simulink model "impedance_subsystem"  (R2023a)
settings: Solver=VariableStepAuto  StartTime=0.0  StopTime=3  RelTol=1e-3
model workspace (MATLAB code in the model file):
  | %% Model component value calculations.
  | % Script recieves Thiele and Small values from mask and then calculates model components' values. It also stores values for sine sweep,
  | % A custom/manual sine sweep was needed inorder to get values for the variable resistors.
  | 
  | Re=         [str2double(get_param('a_LS_model/T&S Values', 'W_Re')), str2double(get_param('a_LS_model/T&S Values', 'T_Re'))];           % The DC resistance of the Voice coil [ohm].
  | 
  | Le=         [str2double(get_param('a_LS_model/T&S Values', 'W_Le')), str2double(get_param('a_LS_model/T&S Values', 'T_Le'))] *1e-3; % The voice coil inductance [H]
  | 
  | 
  | Mms=        [str2double(get_param('a_LS_model/T&S Values', 'W_Mms')), str2double(get_param('a_LS_model/T&S Values', 'T_Mms'))]    *1e-3;  % Mass of the coil and diagphram [Kg]
  | 
  | Sd=         [str2double(get_param('a_LS_model/T&S Values', 'W_Sd')), str2double(get_param('a_LS_model/T&S Values', 'T_Sd'))]    *1e-4;  %Area of diagphram [m^2]
  | Bl=      [str2double(get_param('a_LS_model/T&S Values', 'W_Bl')), str2double(get_param('a_LS_model/T&S Values', 'T_Bl'))];            %The product of magnetic flux density ie Force Factor
  | Vb = [str2double(get_param('a_LS_model/T&S Values', 'Vb')),str2double(get_param('a_LS_model/T&S Values', 'Vb'))];
  | fs =[str2double(get_param('a_LS_model/T&S Values', 'W_fs')),str2double(get_param('a_LS_model/T&S Values', 'T_fs'))];
  | Qes = [str2double(get_param('a_LS_model/T&S Values', 'W_Qes')),str2double(get_param('a_LS_model/T&S Values', 'T_Qes'))];
  | Qms = [str2double(get_param('a_LS_model/T&S Values', 'W_Qms')),str2double(get_param('a_LS_model/T&S Values', 'T_Qms'))];
  | Qts = [str2double(get_param('a_LS_model/T&S Values', 'W_Qts')),str2double(get_param('a_LS_model/T&S Values', 'T_Qts'))];
  | 
  | SweepStart_W_S =str2double(get_param('a_LS_model/Subsystem4', 'SweepStart'));
  | SweepEnd_W_S = str2double(get_param('a_LS_model/Subsystem4', 'SweepStop'));
  | SweepDuration_W_S =str2double(get_param('a_LS_model/Subsystem4', 'SweepTime'));
  | 
  | Vb = Vb ./ 1000;
  | FS = 44100;
  | Qb = 0.707; % Total quality factor
  | 
  | % Constants
  | c = 340; % Speed of sound in m/s
  | rho = 1.2; % Density of air [kg/m^3]
  | 
  | for n = 1:2
  |     alpha(n) = (Qb^2 - Qts(n)^2) / Qts(n)^2;
  |     Rms(n) = (2 * pi * fs(n) * Mms(n)) / Qms(n);
  |     Cms(n) = 1 / (4 * pi^2 * fs(n)^2 * Mms(n));
  |     Vas(n)=rho*c*Sd(n)^2*Cms(n);
  | end
  | 
  | QB = sqrt(alpha(1) + 1) * Qts; % Electroacostics Lecture 4 page 21
  | 
  | for n = 1:2
  | 
  |     r=0.1;
  |     Cab(n) = Vb(n) / (rho * c^2); % Box volume acoustic compliance
  | 
  |     a(n) = sqrt(Sd(n) / pi);
  |     a(n) = 0.85
  |     %Zc(n) = ((rho * c) / Sd(n)) * c; % from grain42n
  | 
  |     Mad(n) = (8 * rho) / (5 * (pi^2) * a(n));% Mad (acoustic mass)
  |     Mar(n)=rho*((a(n)*r)/Sd(n)) % from grain42n
  |     Mad(n)=Mar(n);
  |     Ras(n) = (rho * c) / (pi * (a(n)^2)); %  Ras (acoustic resistance), Beranek page 820/ grain42-page 19
  | 
  |     Lem(n) = Bl(n)^2 * Cms(n); % Lem (driver's equivalent inductance)
  |     Rem(n) = Bl(n)^2 / Rms(n); % Rem (driver's equivalent mechanical resistance),
  |     Cem(n) = Mms(n) / (Bl(n)^2); % Cem (driver's equivalent compliance) from grain41en
  | 
  |     Leb(n) = (Bl(n)/Sd(n))^2 *Cab(n);% Lea (acoustical inductance) grain42-page 19
  |     Rer(n) = (Bl(n)/Sd(n))^2 * 1/Ras(n); % Rea (acoustical resistance)
  |     Cer(n) = (Sd(n)/Bl(n))^2 *Mar(n);%Cea (acoustical compliance
  |     Ced(n) = (Sd(n)/Bl(n))^2 * Mad(n);% Borwick Headphones page 304
  | 
  | end
undefined symbols (not defined in the file): Ced, Cem, Cer, Leb, Lem, Rem
libraries: fl_lib x29, nesl_utility x12, dspsrcs4 x1
settings Model: Creator=Jamie  LastModifiedBy=jamie

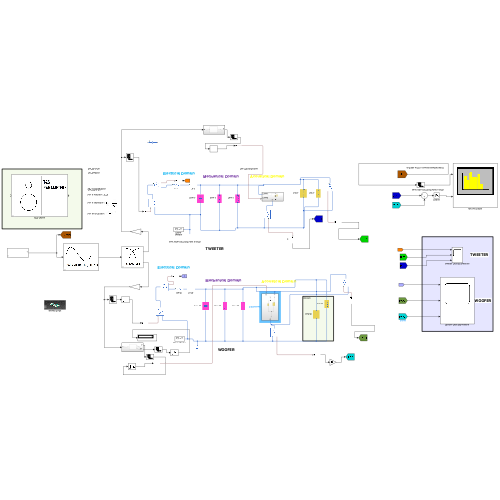
[thumbnail: Simulink's stored preview of the top-level diagram]
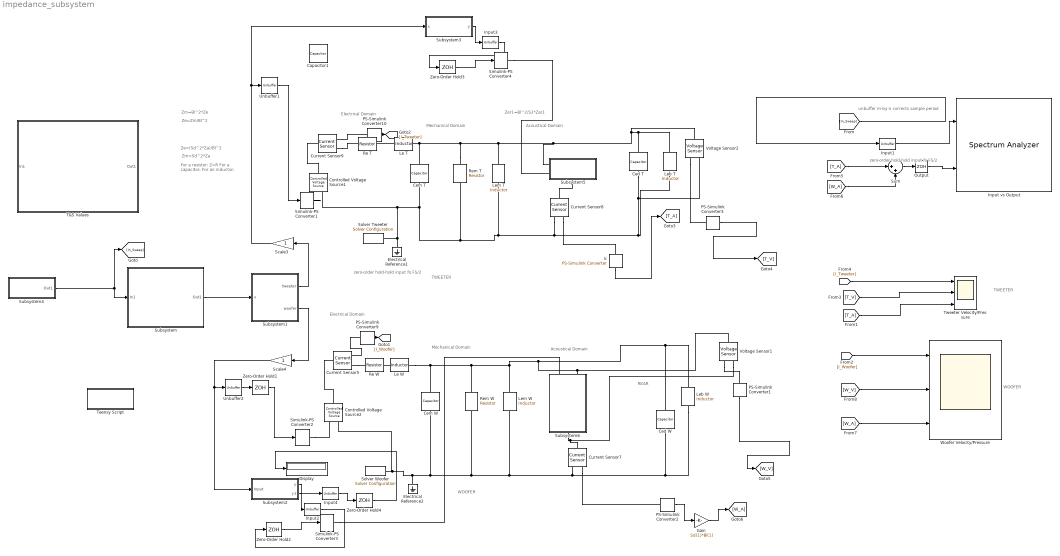
== system impedance_subsystem ==
  note: Zer1=Bl^2/S2*Zar1
  note: Electrical Domain
  note: Mechanical Domain
  note: Mechanical Domain
  note: Zm=Bl^2*Ze
  note: WOOFER
  note: WOOFER
  note: unbuffer m-by-n corrects sample period
  note: TWEETER
  note: Acoustical Domain
  note: zero-order hold-hold input fo FS/2
  note: Zm=Sd^2*Za
  note: For a resistor: Z=R
      | For a capacitor:
      | For an inductor:
  note: zero-order hold-hold input fo FS/2
  note: Ze=Zm/Bl^2
  note: TWEETER
  note: Ze=(Sd^2*Za)/Bl^2
  note: Electrical Domain
  note: Acoustical Domain
  note: REAR
  Capacitor1 : fl_lib/Electrical/Electrical Elements/Capacitor  c=1000 uF  r=1e-6 Ohm  g=0 1/Ohm  i_specify=off  i_priority=None  i=0 A  i_nominal_specify=off  i_nominal_unit=A  i_nominal_value=1  v_specify=off  v_priority=None  v=0 V  v_nominal_specify=off  v_nominal_unit=V  v_nominal_value=1  vc_specify=off  vc_priority=High  vc=0 V  vc_nominal_specify=off  vc_nominal_unit=V  vc_nominal_value=1
  Ced T : fl_lib/Electrical/Electrical Elements/Capacitor  c=Ced(2) F  r=0 Ohm  g=0 1/Ohm  i_specify=off  i_priority=High  i=0 A  i_nominal_specify=off  i_nominal_unit=A  i_nominal_value=1  v_specify=off  v_priority=High  v=0 V  v_nominal_specify=off  v_nominal_unit=V  v_nominal_value=1  vc_specify=off  vc_priority=High  vc=0 V  vc_nominal_specify=off  vc_nominal_unit=V  vc_nominal_value=1
  Ced W : fl_lib/Electrical/Electrical Elements/Capacitor  c=Ced(1) F  r=0 Ohm  g=0 1/Ohm  i_specify=off  i_priority=High  i=0 A  i_nominal_specify=off  i_nominal_unit=A  i_nominal_value=1  v_specify=off  v_priority=High  v=0 V  v_nominal_specify=off  v_nominal_unit=V  v_nominal_value=1  vc_specify=off  vc_priority=High  vc=0 V  vc_nominal_specify=off  vc_nominal_unit=V  vc_nominal_value=1
  Cem T : fl_lib/Electrical/Electrical Elements/Capacitor  c=Cem(2) F  r=0 Ohm  g=0 1/Ohm  i_specify=off  i_priority=High  i=0 A  i_nominal_specify=off  i_nominal_unit=A  i_nominal_value=1  v_specify=off  v_priority=High  v=0 V  v_nominal_specify=off  v_nominal_unit=V  v_nominal_value=1  vc_specify=off  vc_priority=High  vc=0 V  vc_nominal_specify=off  vc_nominal_unit=V  vc_nominal_value=1
  Cem W : fl_lib/Electrical/Electrical Elements/Capacitor  c=Cem(1) F  r=0 Ohm  g=0 1/Ohm  i_specify=off  i_priority=High  i=0 A  i_nominal_specify=off  i_nominal_unit=A  i_nominal_value=1  v_specify=off  v_priority=High  v=0 V  v_nominal_specify=off  v_nominal_unit=V  v_nominal_value=1  vc_specify=off  vc_priority=High  vc=0 V  vc_nominal_specify=off  vc_nominal_unit=V  vc_nominal_value=1
  Controlled Voltage Source1 : fl_lib/Electrical/Electrical Sources/Controlled Voltage Source
  Controlled Voltage Source2 : fl_lib/Electrical/Electrical Sources/Controlled Voltage Source
  Current Sensor{5,7..9} (4 alike) : fl_lib/Electrical/Electrical Sensors/Current Sensor
  Display : Display
  Electrical Reference1 : fl_lib/Electrical/Electrical Elements/Electrical Reference
  Electrical Reference2 : fl_lib/Electrical/Electrical Elements/Electrical Reference
  Gain : Gain  Gain=Sd(1)*Bl(1)
  "Input vs Output " : SpectrumAnalyzer  NumInputPorts=2  WindowPosition=[115.000000,110.000000,1536.000000,801.000000,]  ScopeFrameLocation=window  SpectrumType=Power density  Method=Welch  SampleRate=48000  PlotAsTwoSidedSpectrum=off  FrequencyScale=Log  AxesScaling=Manual  FrequencySpan=Start and stop frequencies  StartFrequency=4000  StopFrequency=20e3  AveragingMethod=Exponential  ForgettingFactor=0.4  SpectrumUnits=dBm/Hz  PlotMaxHoldTrace=on  YLimits=[-240.83457972,36.18497741]  ShowLegend=on  SelectedToolstripTab=spectrumAnalyzerToolstrip.spectrumTab  MeasurementChannel=4
      settings: OpenAtSimulationStart=off
  Input{1..4} (4 alike) : Unbuffer
  Le T : fl_lib/Electrical/Electrical Elements/Inductor  l=Le(2) H  r=0 Ohm  g=0 1/Ohm  i_specify=off  i_priority=High  i=0 A  i_nominal_specify=off  i_nominal_unit=A  i_nominal_value=1  v_specify=off  v_priority=High  v=0 V  v_nominal_specify=off  v_nominal_unit=V  v_nominal_value=1  i_L_specify=off  i_L_priority=High  i_L=0 A  i_L_nominal_specify=off  i_L_nominal_unit=A  i_L_nominal_value=1
  Le W : fl_lib/Electrical/Electrical Elements/Inductor  l=Le(1) H  r=0 Ohm  g=0 1/Ohm  i_specify=off  i_priority=High  i=0 A  i_nominal_specify=off  i_nominal_unit=A  i_nominal_value=1  v_specify=off  v_priority=High  v=0 V  v_nominal_specify=off  v_nominal_unit=V  v_nominal_value=1  i_L_specify=off  i_L_priority=High  i_L=0 A  i_L_nominal_specify=off  i_L_nominal_unit=A  i_L_nominal_value=1
  Leb T : fl_lib/Electrical/Electrical Elements/Inductor  l=Leb(2) H  r=0 Ohm  g=0 1/Ohm  i_specify=off  i_priority=High  i=0 A  i_nominal_specify=off  i_nominal_unit=A  i_nominal_value=1  v_specify=off  v_priority=High  v=0 V  v_nominal_specify=off  v_nominal_unit=V  v_nominal_value=1  i_L_specify=off  i_L_priority=High  i_L=0 A  i_L_nominal_specify=off  i_L_nominal_unit=A  i_L_nominal_value=1
  Leb W : fl_lib/Electrical/Electrical Elements/Inductor  l=Leb(1) H  r=0 Ohm  g=0 1/Ohm  i_specify=off  i_priority=High  i=0 A  i_nominal_specify=off  i_nominal_unit=A  i_nominal_value=1  v_specify=off  v_priority=High  v=0 V  v_nominal_specify=off  v_nominal_unit=V  v_nominal_value=1  i_L_specify=off  i_L_priority=High  i_L=0 A  i_L_nominal_specify=off  i_L_nominal_unit=A  i_L_nominal_value=1
  Lem T : fl_lib/Electrical/Electrical Elements/Inductor  l=Lem(2) H  r=0 Ohm  g=0 1/Ohm  i_specify=off  i_priority=High  i=0 A  i_nominal_specify=off  i_nominal_unit=A  i_nominal_value=1  v_specify=off  v_priority=High  v=0 V  v_nominal_specify=off  v_nominal_unit=V  v_nominal_value=1  i_L_specify=off  i_L_priority=High  i_L=0 A  i_L_nominal_specify=off  i_L_nominal_unit=A  i_L_nominal_value=1
  Lem W : fl_lib/Electrical/Electrical Elements/Inductor  l=Lem(1) H  r=0 Ohm  g=0 1/Ohm  i_specify=off  i_priority=High  i=0 A  i_nominal_specify=off  i_nominal_unit=A  i_nominal_value=1  v_specify=off  v_priority=High  v=0 V  v_nominal_specify=off  v_nominal_unit=V  v_nominal_value=1  i_L_specify=off  i_L_priority=High  i_L=0 A  i_L_nominal_specify=off  i_L_nominal_unit=A  i_L_nominal_value=1
  Output : ZeroOrderHold  SampleTime=1/FS
  PS-Simulink Converter{1..3,9..10} (5 alike) : nesl_utility/PS-Simulink Converter  PhysicalDomain=network_engine_domain  SubClassName=ps_output  LeftPortType=input  RightPortType=output  PseudoPeriodic=off  Frequencies=[]  VectorFormat=1-D array  Unit=1  AffineConversion=off
  Re T : fl_lib/Electrical/Electrical Elements/Resistor  R=Re(2) Ohm  i_specify=off  i_priority=High  i=0 A  i_nominal_specify=off  i_nominal_unit=A  i_nominal_value=1  v_specify=off  v_priority=High  v=0 V  v_nominal_specify=off  v_nominal_unit=V  v_nominal_value=1
  Re W : fl_lib/Electrical/Electrical Elements/Resistor  R=Re(1) Ohm  i_specify=off  i_priority=High  i=0 A  i_nominal_specify=off  i_nominal_unit=A  i_nominal_value=1  v_specify=off  v_priority=High  v=0 V  v_nominal_specify=off  v_nominal_unit=V  v_nominal_value=1
  Rem T : fl_lib/Electrical/Electrical Elements/Resistor  R=Rem(2) Ohm  i_specify=off  i_priority=High  i=0 A  i_nominal_specify=off  i_nominal_unit=A  i_nominal_value=1  v_specify=off  v_priority=High  v=0 V  v_nominal_specify=off  v_nominal_unit=V  v_nominal_value=1
  Rem W : fl_lib/Electrical/Electrical Elements/Resistor  R=Rem(1) Ohm  i_specify=off  i_priority=High  i=0 A  i_nominal_specify=off  i_nominal_unit=A  i_nominal_value=1  v_specify=off  v_priority=High  v=0 V  v_nominal_specify=off  v_nominal_unit=V  v_nominal_value=1
  Scale3 : Gain
  Scale4 : Gain
  Simulink-PS Converter{1..4} (4 alike) : nesl_utility/Simulink-PS Converter  PhysicalDomain=network_engine_domain  SubClassName=ps_input  LeftPortType=input  RightPortType=output  PseudoPeriodic=off  Frequencies=[]  NoiseDistribution=none  NoiseParameters=[]  Unit=1  AffineConversion=off  FilteringAndDerivatives=zero  SimscapeFilterOrder=1  InputFilterTimeConstant=0.001  UdotUserProvided=1
  Solver Tweeter : nesl_utility/Solver Configuration  PhysicalDomain=network_engine_domain  SubClassName=solver  LeftPortType=input  RightPortType=generic  Tones=[]  Harmonics=[]  SimulateNoise=off  Profile=off  UseLocalSampling=off  EnableSwitchedLinearOptims=on  FrequencyDomain=off  UseCCode=off  RelTol=0.001  AbsTol=1e-06  MinStep=1e-09  ToWorkspace=off  RevertToSquareIcSolve=off  NumHomotopyIterations=100  PhasorMode=off  PhasorModeNumHarmonics=1  ConsistencySolver=NEWTON_FTOL  IndexReductionMethod=DerivativeReplacement  DoDC=off  ResidualTolerance=1e-09  ConsistencyTolSource=GLOBAL  ConsistencyAbsTol=0.001  ConsistencyRelTol=0.001  ConsistencyTolFactor=0.001  UseLocalSolver=off  LocalSolverChoice=NE_BACKWARD_EULER_ADVANCER  ResolveIndetEquations=on  FunctionEvalNumThread=1  LocalSolverSampleTime=0.001  DoFixedCost=off  MaxNonlinIter=3  MaxModeIter=2  ComputeImpulses=off  ImpulseIterations=2  LinearAlgebra=Sparse  LinearAlgebraNumThread=0  EquationFormulation=NE_TIME_EF  DelaysMemoryBudget=1024  AutomaticFiltering=on  FilteringTimeConstant=0.001  PartitionStorageMethod=AS_NEEDED  PartitionMemoryBudget=1024  PartitionMethod=FAST
  "Solver Woofer " : nesl_utility/Solver Configuration  PhysicalDomain=network_engine_domain  SubClassName=solver  LeftPortType=input  RightPortType=generic  Tones=[]  Harmonics=[]  SimulateNoise=off  Profile=off  UseLocalSampling=off  EnableSwitchedLinearOptims=on  FrequencyDomain=off  UseCCode=off  RelTol=0.001  AbsTol=1e-06  MinStep=1e-09  ToWorkspace=off  RevertToSquareIcSolve=off  NumHomotopyIterations=100  PhasorMode=off  PhasorModeNumHarmonics=1  ConsistencySolver=NEWTON_FTOL  IndexReductionMethod=DerivativeReplacement  DoDC=off  ResidualTolerance=1e-09  ConsistencyTolSource=GLOBAL  ConsistencyAbsTol=0.001  ConsistencyRelTol=0.001  ConsistencyTolFactor=0.001  UseLocalSolver=off  LocalSolverChoice=NE_BACKWARD_EULER_ADVANCER  ResolveIndetEquations=on  FunctionEvalNumThread=1  LocalSolverSampleTime=0.001  DoFixedCost=off  MaxNonlinIter=3  MaxModeIter=2  ComputeImpulses=off  ImpulseIterations=2  LinearAlgebra=Sparse  LinearAlgebraNumThread=0  EquationFormulation=NE_TIME_EF  DelaysMemoryBudget=1024  AutomaticFiltering=on  FilteringTimeConstant=0.001  PartitionStorageMethod=AS_NEEDED  PartitionMemoryBudget=1024  PartitionMethod=FAST
  Subsystem : Subsystem  mask{plotFlag=on, BW1=88.120, GdB1=0, FC1=500, BW2=59.410, GdB2=0, FC2=1.352e+03, BW3=100.0, GdB3=0, FC3=400, BW4=67.330, GdB4=0, FC4=400, BW5=66.340, GdB5=0, FC5=129.131, BW6=53.470, GdB6=0, FC6=833.739}
      mask prompts: plotFlag "Plot EQ response"; BW1 "Band Width 1"; GdB1 "Gain 1"; FC1 "Center Frequency 1"; BW2 "Band Width 2"; GdB2 "Gain 2"; FC2 "Center Frequency 2"; BW3 "Band Width 3"; GdB3 "Gain 3"; FC3 "Center Frequency 3"; BW4 "Band Width 4"; GdB4 "Gain 4"; FC4 "Center Frequency 4"; BW5 "Band Width 5"; GdB5 "Gain 5"; FC5 "Center Frequency 5"; BW6 "Band Width 6"; GdB6 "Gain 6"; FC6 "Center Frequency 6"
      mask DialogControl DescTextVar Prompt: Highest and lowest fc will be shelving
      mask Display: image('parametric equalizer.jpg'); % Use "Edit Image" on toolstrip to change.
  Subsystem1 : Subsystem  mask{fc=1.069e+03, G_T=5.040, G_W=0, response=on}
      mask prompts: G_T "Tweeter Gain"; G_W "Wooofer Gain"; response "Plot frequency response"
      mask Display: image('crossover.jpg'); % Use "Edit Image" on toolstrip to change.
  Subsystem2 : Subsystem
  Subsystem3 : Subsystem
  Subsystem4 : Subsystem  mask{SweepStart=20.0, SweepStop=2.000e+04, SweepTime=3}
      mask prompts: SweepStart "Sweep start frequency"; SweepStop "Sweep end frequency"; SweepTime "Sweep time in seconds"
  Subsystem5 : Subsystem
      settings: PortSchema="{\"entries\":[{\"content\":{\"sides\":[{\"content\":{\"connectorIds\":[\"LConn1\",\"LConn2\"]},\"type\":\"ConnectorPlacement.EquallySpacedRectSide\",\"uuid\":\"25cb09ee-3296-462f-b9af-d61a9c9e7aa7\"},{\"content\":{\"side\":\"RIGHT\"},\"type\":\"ConnectorPlacement.EquallySpacedRectSide\",\"uuid\":\"56b7f4d6-4575-4235-9b40-81966edcf44f\"},{\"content\":{\"side\":\"TOP\"},\"type\":\"ConnectorPlacement.EquallySpacedRectSide\",\"uuid\":\"6b15c573-0474-440b-b33a-e36954ffc872\"},{\"content\":{\"connectorIds\":[\"RConn1\"],\"side\":\"BOTTOM\"},\"type\":\"ConnectorPlacement.EquallySpacedRectSide\",\"uuid\":\"46e98950-34e6-48c0-ad9b-f72df4e485f9\"}]},\"type\":\"ConnectorPlacement.EquallySpacedConnector\",\"uuid\":\"8a04249c-d482-4767-9f60-a5a89d31e022\"}],\"packageUris\":[\"http://schema.mathworks.com/mf0/Connector/R2020b\"],\"version\":\"1.0\"}"
  Subsystem6 : Subsystem
  Sum : Sum  Inputs=|++
  T&S Values : Subsystem  mask{Vb=1000, W_Sd=56.4, T_Sd=6.2, W_Re=3.7, T_Re=3.2, W_Le=0.22, T_Le=0.04, W_Bl=5, T_Bl=1.6, W_Mms=6.7, T_Mms=0.3, W_fs=74.6, T_fs=750, W_Qts=4.84, T_Qts=1.12, W_Qes=0.47, T_Qes=1.78, W_Qms=0.43, T_Qms=3.0}
      mask prompts: Vb "Box Volume"; W_Sd "Woofer Sd"; T_Sd "Tweeter Sd"; W_Re "Woofer Re"; T_Re "Tweeter Re"; W_Le "Woofer Le"; T_Le "Tweeter Le"; W_Bl "Woofer Bl"; T_Bl "Tweeter Bl"; W_Mms "Woofer Mms"; T_Mms "Tweeter Mms"; W_fs "Woofer fs"; T_fs "Tweeter fs"; W_Qts "Woofer Qts"; T_Qts "Tweeter Qts"; W_Qes "Woofer Qes"; T_Qes "Tweeter Qes"; W_Qms "Woofer Qms"; T_Qms "Tweeter Qms"
      mask Display: image('$imagefile'); % Use "Edit Image" on toolstrip to change.
  Teensy Script : Subsystem  mask{savename=modified_script2.txt}
      mask prompts: savename "Script.txt save name"
      mask Display: image('teensy_pic_for_mask.jpg'); % Use "Edit Image" on toolstrip to change.
  Tweeter Velocity/Pressure : Scope  NumInputPorts=3
  Unbuffer1 : Unbuffer
  Unbuffer2 : Unbuffer
  Voltage Sensor1 : fl_lib/Electrical/Electrical Sensors/Voltage Sensor
  Voltage Sensor2 : fl_lib/Electrical/Electrical Sensors/Voltage Sensor
  Woofer Velocity/Pressure : Scope  NumInputPorts=3
  Zero-Order Hold{1..4} (4 alike) : ZeroOrderHold  SampleTime=1/FS
  "k " : nesl_utility/PS-Simulink Converter  PhysicalDomain=network_engine_domain  SubClassName=ps_output  LeftPortType=input  RightPortType=output  PseudoPeriodic=off  Frequencies=[]  VectorFormat=1-D array  Unit=1  AffineConversion=off
  wires:
  Zero-Order Hold3/1 -> Simulink-PS Converter4/1
  Subsystem2/1(y) -> Input2/1
  Zero-Order Hold1/1 -> Simulink-PS Converter2/1
  [I_Tweeter] -> Tweeter Velocity/Pressure/1
  PS-Simulink Converter9/1 -> [I_Woofer]
  Subsystem3/1(y) -> Input3/1
  Input2/1 -> Zero-Order Hold2/1
  Subsystem1/2(woofer) -> Scale4/1
  Unbuffer2/1 -> Zero-Order Hold1/1
  Zero-Order Hold2/1 -> Simulink-PS Converter3/1
  PS-Simulink Converter3/1 -> [T_V]
  Input3/1 -> Zero-Order Hold3/1
  [I_Woofer] -> Woofer Velocity/Pressure/1
  [T_A] -> Sum/1
  PS-Simulink Converter10/1 -> [I_Tweeter]
  Subsystem4/1(Out1) -> [In_Sweep], Subsystem/1(In1)
  Sum/1 -> Output/1
  Unbuffer1/1 -> Simulink-PS Converter1/1
  Subsystem1/1(tweeter) -> Scale3/1
  "k "/1 -> [T_A]
  [W_A] -> Sum/2
  PS-Simulink Converter1/1 -> [W_V]
  Subsystem/1(Out1) -> Subsystem1/1(x)
  Subsystem2/2(y1) -> Input4/1
  Input4/1 -> Zero-Order Hold4/1
  Zero-Order Hold4/1 -> Display/1
  Input1/1 -> "Input vs Output "/1
  [In_Sweep] -> Input1/1
  Output/1 -> "Input vs Output "/2
  Scale3/1 -> Subsystem3/1(x), Unbuffer1/1
  Scale4/1 -> Subsystem2/1(Input), Unbuffer2/1
  PS-Simulink Converter2/1 -> Gain/1
  Gain/1 -> [W_A]
  [W_V] -> Woofer Velocity/Pressure/2
  [W_A] -> Woofer Velocity/Pressure/3
  [T_A] -> Tweeter Velocity/Pressure/3
  [T_V] -> Tweeter Velocity/Pressure/2
  connections:
  Rem T/LConn1 -- Cem T/LConn1 -- Le T/RConn1 -- Lem T/LConn1 -- Subsystem5/LConn1 -- Ced T/LConn1 -- Leb T/LConn1 -- Voltage Sensor2/LConn1
  Lem W/LConn1 -- Voltage Sensor1/LConn1 -- Subsystem6/LConn1 -- Ced W/LConn1 -- Leb W/LConn1 -- Rem W/LConn1 -- Cem W/LConn1 -- Le W/RConn1
  Voltage Sensor1/RConn1 -- PS-Simulink Converter1/LConn1
  Simulink-PS Converter1/RConn1 -- Controlled Voltage Source1/RConn1
  Simulink-PS Converter4/RConn1 -- Subsystem5/LConn2
  PS-Simulink Converter10/LConn1 -- Current Sensor9/RConn1
  Ced W/RConn1 -- Current Sensor7/RConn2 -- "Solver Woofer "/RConn1 -- Controlled Voltage Source2/RConn2 -- Electrical Reference2/LConn1 -- Cem W/RConn1 -- Rem W/RConn1 -- Lem W/RConn1 -- Leb W/RConn1
  Le W/LConn1 -- Re W/RConn1
  Current Sensor8/RConn1 -- "k "/LConn1
  Simulink-PS Converter2/RConn1 -- Controlled Voltage Source2/RConn1
  Simulink-PS Converter3/RConn1 -- Subsystem6/LConn2
  Le T/LConn1 -- Re T/RConn1
  Ced T/RConn1 -- Voltage Sensor2/RConn2 -- Current Sensor8/RConn2 -- Lem T/RConn1 -- Rem T/RConn1 -- Solver Tweeter/RConn1 -- Electrical Reference1/LConn1 -- Controlled Voltage Source1/RConn2 -- Cem T/RConn1 -- Leb T/RConn1
  PS-Simulink Converter9/LConn1 -- Current Sensor5/RConn1
  Voltage Sensor2/RConn1 -- PS-Simulink Converter3/LConn1
  Current Sensor7/RConn1 -- PS-Simulink Converter2/LConn1
  Current Sensor9/RConn2 -- Re T/LConn1
  Current Sensor9/LConn1 -- Controlled Voltage Source1/LConn1
  Controlled Voltage Source2/LConn1 -- Current Sensor5/LConn1
  Current Sensor5/RConn2 -- Re W/LConn1
  Subsystem5/RConn1 -- Current Sensor8/LConn1
  Subsystem6/RConn1 -- Current Sensor7/LConn1 -- Voltage Sensor1/RConn2

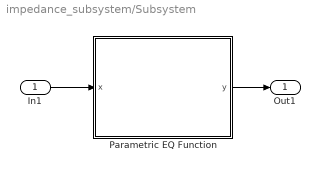
== system impedance_subsystem/Subsystem ==
  In1 : Inport
  Parametric EQ Function : MATLAB Function  TreatAsAtomicUnit=on
  Out1 : Outport
  wires:
  In1/1 -> Parametric EQ Function/1(x)
  Parametric EQ Function/1(y) -> Out1/1

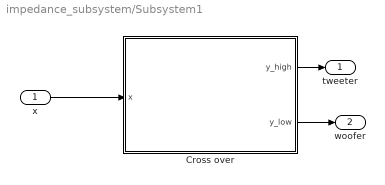
== system impedance_subsystem/Subsystem1 ==
  x : Inport
  Cross over : MATLAB Function  TreatAsAtomicUnit=on
  tweeter : Outport
  woofer : Outport  Port=2
  wires:
  x/1 -> Cross over/1(x)
  Cross over/1(y_high) -> tweeter/1
  Cross over/2(y_low) -> woofer/1

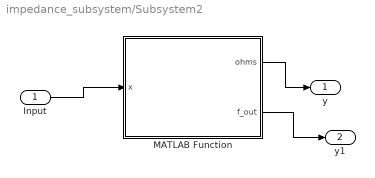
== system impedance_subsystem/Subsystem2 ==
  Input : Inport
  MATLAB Function : MATLAB Function  TreatAsAtomicUnit=on
  y : Outport
  y1 : Outport  Port=2
  wires:
  MATLAB Function/1(ohms) -> y/1
  MATLAB Function/2(f_out) -> y1/1
  Input/1 -> MATLAB Function/1(x)

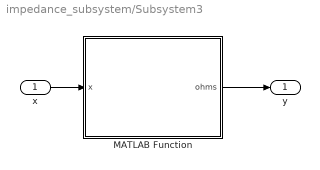
== system impedance_subsystem/Subsystem3 ==
  x : Inport
  MATLAB Function : MATLAB Function  TreatAsAtomicUnit=on
  y : Outport
  wires:
  x/1 -> MATLAB Function/1(x)
  MATLAB Function/1(ohms) -> y/1

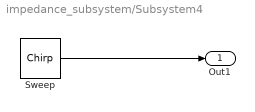
== system impedance_subsystem/Subsystem4 ==
  Sweep : dspsrcs4/Chirp  sweep=Logarithmic  mode=Unidirectional  f0=SweepStart  f1=SweepStop  t1=SweepTime  Tsweep=SweepTime  phase=0  Ts=1/FS  spf=1024  datatype=Double  OutputFrames=off
  Out1 : Outport
  wires:
  Sweep/1 -> Out1/1

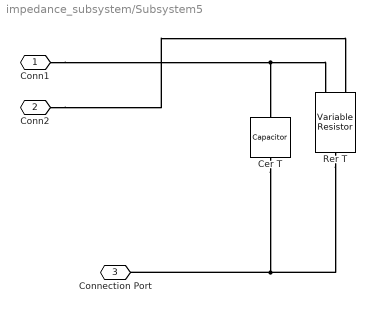
== system impedance_subsystem/Subsystem5 ==
  Cer T : fl_lib/Electrical/Electrical Elements/Capacitor  c=Cer(2) F  r=0 Ohm  g=0 1/Ohm  i_specify=off  i_priority=High  i=0 A  i_nominal_specify=off  i_nominal_unit=A  i_nominal_value=1  v_specify=off  v_priority=High  v=0 V  v_nominal_specify=off  v_nominal_unit=V  v_nominal_value=1  vc_specify=off  vc_priority=High  vc=0 V  vc_nominal_specify=off  vc_nominal_unit=V  vc_nominal_value=1
  Rer T : fl_lib/Electrical/Electrical Elements/Variable Resistor  Rmin=0 Ohm  i_specify=off  i_priority=None  i=0 A  i_nominal_specify=off  i_nominal_unit=A  i_nominal_value=1  v_specify=off  v_priority=None  v=0 V  v_nominal_specify=off  v_nominal_unit=V  v_nominal_value=1
  Conn1 : PMIOPort  Side=Left
  Conn2 : PMIOPort  Port=2  Side=Left
  Connection Port : PMIOPort  Port=3  Side=Right
  connections:
  Conn1/RConn1 -- Rer T/LConn2 -- Cer T/LConn1
  Cer T/RConn1 -- Rer T/RConn1 -- Connection Port/RConn1
  Conn2/RConn1 -- Rer T/LConn1

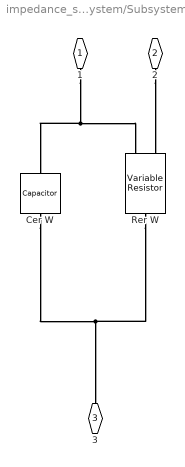
== system impedance_subsystem/Subsystem6 ==
  Cer W : fl_lib/Electrical/Electrical Elements/Capacitor  c=Cer(1) F  r=0 Ohm  g=0 1/Ohm  i_specify=off  i_priority=High  i=0 A  i_nominal_specify=off  i_nominal_unit=A  i_nominal_value=1  v_specify=off  v_priority=High  v=0 V  v_nominal_specify=off  v_nominal_unit=V  v_nominal_value=1  vc_specify=off  vc_priority=High  vc=0 V  vc_nominal_specify=off  vc_nominal_unit=V  vc_nominal_value=1
  Rer W : fl_lib/Electrical/Electrical Elements/Variable Resistor  Rmin=0 Ohm  i_specify=off  i_priority=None  i=0 A  i_nominal_specify=off  i_nominal_unit=A  i_nominal_value=1  v_specify=off  v_priority=None  v=0 V  v_nominal_specify=off  v_nominal_unit=V  v_nominal_value=1
  1 : PMIOPort  Side=Left
  2 : PMIOPort  Port=2  Side=Left
  3 : PMIOPort  Port=3  Side=Right
  connections:
  Cer W/RConn1 -- Rer W/RConn1 -- 3/RConn1
  2/RConn1 -- Rer W/LConn1
  1/RConn1 -- Cer W/LConn1 -- Rer W/LConn2

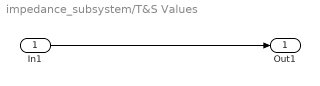
== system impedance_subsystem/T&S Values ==
  In1 : Inport
  Out1 : Outport
  wires:
  In1/1 -> Out1/1

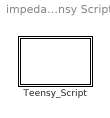
== system impedance_subsystem/Teensy Script ==
  Teensy_Script : MATLAB Function  TreatAsAtomicUnit=on

== matlab function impedance_subsystem/Subsystem1/Cross over ==
  data: x input; y_high output; y_low output
%% Linkwitz and Riley Crossover function that recieves user parameters from Simulink mask

function [y_high,y_low]= crossover(x)

persistent zi_low_1 % Persistent filter states held over for next block 
persistent zi_low_2
persistent zi_high_1
persistent zi_high_2

persistent flag             % flags for parts of code that only need to be run once to improve code efficiency 
persistent counter
persistent plotFlag 

if isempty(flag)
    flag=1;
end

coder.extrinsic('get_param') %coder.entrinsic allows for functions to be surported in simulink that would otherwise not be
coder.extrinsic('xticks')
coder.extrinsic('xticklabels')
coder.extrinsic("assignin")
coder.extrinsic("evalin")
coder.extrinsic("sgtitle")


plotFlag = get_param('a_LS_model/Subsystem1', 'response');


if isempty(counter)
      counter=0;
end

fs=double(44100);

% Getting user input from mask

G_T = str2double(get_param('a_LS_model/Subsystem1', 'G_T'));
G_W = str2double(get_param('a_LS_model/Subsystem1', 'G_W'));

if flag==1
fc = str2double(get_param('a_LS_model/Subsystem1', 'fc'));

H=zeros(512,1);
w=double(0);

w =fc/(fs/2);

y_high=zeros(length(x),1);
y_low=zeros(length(x),1);

[B_low, A_low]= butter(2, w, "low");

[B_high, A_high]= butter(2, w, "high");
            
disp('A HIGH')
disp(A_high)

assignin('base', 'B_Low_shel', B_low); % Assign to base for use in teensy script writing also speeds code as can be read rather than calulated for every block but first.
assignin('base', 'A_Low_shel', A_low);

assignin('base', 'B_High_shel', B_high);
assignin('base', 'A_High_shel', A_high);

flag=2;

else

    A_high = evalin('base', 'A_High_shel'); % Read from base rather than calculate again for faster code
    A_low = evalin('base', 'A_Low_shel');

    B_high = evalin('base', 'B_High_shel');
    B_low = evalin('base', 'B_Low_shel');

end


%%%%%%%%%%%%%%%%%%%%%%%%%%%%%%%%%%%%%%%%%%%%%%%%%%%%%%%%%%%%%%%%%%%%%%
%% Low pass
   x_low=x;
   if isempty (zi_low_1)
    zi_low_1=zeros(3,1);
    zi_low_2=zeros(3,1);
    zi_high_1=zeros(3,1);
    zi_high_2=zeros(3,1);
   end
   

           [y_low, zi_low_1]=myFilter(B_low,A_low,x_low,zi_low_1);

           x_low=y_low;
     

           [y_low, zi_low_2]=myFilter(B_low,A_low,x_low, zi_low_2);
           
           


           
%%%%%%%%%%%%%%%%%%%%%%%%%%%%%%%%%%%%%%%%%%%%%%%%%%%%%%%%%%%%%%%
%% High pass
   
   
        x_high=x;
        zi_high=[0,0];
          
          
          [y_high, zi_high_1]=myFilter(B_high,A_high,x_high,zi_high_1);
           
           x_high=y_high;
         
           
           [y_high, zi_high_2]=myFilter(B_high,A_high,x_high,zi_high_2);


y_high=y_high*(10^(G_T/20));
y_low=y_low*(10^(G_W/20));

    
%% Plotting

if counter == 0 && strcmp(plotFlag,'on')
        figure(2)

        [H_high, ~]=freqz(B_high,A_high);
        [H_low, w]=freqz(B_low,A_low);


        f=w/(2*pi)*fs;

        H_high=H_high.*H_high;

        H_low=H_low.*H_low;

        subplot(3,1,1)
        semilogx(f, mag2db(abs(H_high)));
        xlabel('Frequency (Hz)')
        ylabel('Magnitude (dB)')
        title('Magnitude Response High Pass')
        ylim([-14 14])
        xlim([min(f) max(f)])
        disp(f)
        xticks([(min(f)+20) 62.5 125 250 500 1000 2000 4000 8000 16000])
        xticklabels({'20','62.5','125','250','500','1000','2000','4K','8K','16K'})

        subplot(3,1,2)
        semilogx(f, mag2db(abs(H_low)));
        xlabel('Frequency (Hz)')
        ylabel('Magnitude (dB)')
        title('Magnitude Response Low pass')
        ylim([-14 14])
        xlim([min(f) max(f)])
        disp(f)
        xticks([(min(f)+20) 62.5 125 250 500 1000 2000 4000 8000 16000])
        xticklabels({'20','62.5','125','250','500','1000','2000','4K','8K','16K'})
        hold on
        subplot(3,1,3)
        semilogx(f, mag2db(abs(H_low)));
        semilogx(f, mag2db(abs(H_high)));
        semilogx(f, mag2db(abs(H_high+H_low)));
        xlabel('Frequency (Hz)')
        ylabel('Magnitude (dB)')
        title('Magnitude Response Linkwitz-Riley')
        ylim([-14 14])
        xlim([min(f) max(f)])
        disp(f)
        xticks([(min(f)+20) 62.5 125 250 500 1000 2000 4000 8000 16000])
        xticklabels({'20','62.5','125','250','500','1000','2000','4K','8K','16K'})
        
        sgtitle('Crossover');
        
        
end


counter=counter+1

        
end


%%%%%%%%%%%%%%%%%%%%%%%%%%%%%%%%%%%%%%%%%%%%%
%% filter function
function [y, zf] = myFilter(B, A, x,zi)


count=double(0);
b0=double(B(1));
b1=double(B(2));
b2=double(B(3));
a0=double(A(1));
a1=double(A(2));
a2=double(A(3));


y = ones(length(x),1);

for n = 1:length(x)
    

    y(n) = (b0/a0) * x(n) + zi(1);
    
    zi(1) = (b1/a0) * x(n) + zi(2) - (a1/a0) * y(n);
   
    zi(2) = (b2/a0) * x(n) + zi(3) - (a2/a0) * y(n);
    
count = count+1;
end



zf = zi;

end

== matlab function impedance_subsystem/Subsystem/Parametric EQ Function ==
  data: x input; y output

function y=paramFunc(x)

coder.extrinsic('get_param')
coder.extrinsic('xticks')
coder.extrinsic('xticklabels')
coder.extrinsic('assignin')
coder.extrinsic('evalin')
coder.extrinsic("sgtitle")

persistent zi_Arr
persistent plotFlag 
persistent counter
persistent coeff_flag


if isempty(coeff_flag)
      coeff_flag=1;
end

if isempty(counter)
      counter=0;
end

counter=counter+1;
fs=44100;

%%
%%%%%%%%%%%%%%%%%%%%%%%%%%%%%%%%%%%%%%%%%%%%%%%%%%%%%%%%%%%%%%%%%%%%%%%%%%%%%%%%%%%%%%%%%%%%%%%%%%%%%%%%%%%%%%%%%%%%%%%%%%%%%%%%%%%%




Numband=double(6);

V0=zeros(Numband,1);
V0_peq=zeros(Numband,1);
K= zeros(Numband,1);
fc=zeros(Numband,1);
BWp=zeros(Numband,1);
BW=zeros(Numband,1);
N=zeros(Numband,1);
w0=zeros(Numband,1);
gain= zeros(Numband,1);
H=complex(ones(512,1));
H_temp=complex(ones(512,Numband));

plotFlag = get_param('a_LS_model/Subsystem', 'plotFlag');
if coeff_flag==1
    
gain(1) = str2double(get_param('a_LS_model/Subsystem', 'GdB1'));
gain(2) = str2double(get_param('a_LS_model/Subsystem', 'GdB2'));
gain(3) = str2double(get_param('a_LS_model/Subsystem', 'GdB3'));
gain(4) = str2double(get_param('a_LS_model/Subsystem', 'GdB4'));
gain(5) = str2double(get_param('a_LS_model/Subsystem', 'GdB5'));
gain(6) = str2double(get_param('a_LS_model/Subsystem', 'GdB6'));



fc(1) = str2double(get_param('a_LS_model/Subsystem', 'FC1'));
fc(2) = str2double(get_param('a_LS_model/Subsystem', 'FC2'));
fc(3) = str2double(get_param('a_LS_model/Subsystem', 'FC3'));
fc(4) = str2double(get_param('a_LS_model/Subsystem', 'FC4'));
fc(5) = str2double(get_param('a_LS_model/Subsystem', 'FC5'));
fc(6) = str2double(get_param('a_LS_model/Subsystem', 'FC6'));


BWp(1) = str2double(get_param('a_LS_model/Subsystem', 'BW1'));
BWp(2) = str2double(get_param('a_LS_model/Subsystem', 'BW2'));
BWp(3) = str2double(get_param('a_LS_model/Subsystem', 'BW3'));
BWp(4) = str2double(get_param('a_LS_model/Subsystem', 'BW4'));
BWp(5) = str2double(get_param('a_LS_model/Subsystem', 'BW5'));
BWp(6) = str2double(get_param('a_LS_model/Subsystem', 'BW6'));

Filt=zeros(Numband,4);
b0=double(0);
b1=double(0);
b2=double(0);
a0=double(0);
a1=double(0);
a2=double(0);

for i=1:Numband
 
Filt(i,1)= gain(i);
Filt(i,2)=fc(i);
Filt(i,3)=BWp(i);
Filt(i,4)=BWp(i)*gain(i);
end

minFc=min(Filt(1:end,2));
maxFc=max(Filt(1:end,2));



for i=1:Numband
V0(i)= 10^(Filt(i,1)/20);%For shelving filters  
    K(i)= tan ((pi*fc(i))/fs);
    
    V0_peq(i)=Filt(i,1);%For peaking filter
    w0(i) = Filt(i,2)/(fs/2); 
    N=double(2);


    y=zeros(length(x),1);
   
    BW(i)=(Filt(i,2)*Filt(i,3))/100;%percentage of fc to Hz
    BW(i)=BW(i)/(fs/2);
    
end

[B,A] = designParamEQ(2,V0_peq',w0', BW','Orientation','row');



for i=1:Numband


        if Filt(i,2) ==minFc && V0(i)>0
            %Low Shelf Boost
            b0 = ((1)+(sqrt(2*V0(i))*K(i))+V0(i)*K(i)^2) / ((1)+(sqrt(2)*K(i))+K(i)^2);
            b1 = ((2)*(V0(i)*(K(i)^2)-1)) / ((1)+(sqrt(2)*K(i))+K(i)^2);
            b2 = ((1)-(sqrt(2*V0(i))*K(i))+V0(i)*K(i)^2) / ((1)+(sqrt(2)*K(i))+K(i)^2);
            a0 = 1;
            a1 =  ((2)*((K(i)^2)-1)) / ((1)+(sqrt(2)*K(i))+K(i)^2);
            a2 = ((1)-sqrt(2)*K(i)+K(i)^2) / ((1)+(sqrt(2)*K(i))+K(i)^2);

            B(i,:)=[b0,b1,b2];
            A(i,:)=[a0,a1,a2];


        elseif Filt(i,2) == minFc && V0(i)<0
            %Low Shelf Cut


            b0=(V0(i)*(1+sqrt(2)*K(i)+K(i)^2)) / (V0(i)+sqrt(2*V0(i))*K(i)+K(i)^2);
            b1=(2*V0(i)*(K(i)^2-1)) / (V0(i)+sqrt(2*V0(i))*K(i)+K(i)^2);
            b2=(V0(i)*(1-sqrt(2)*K(i)+K(i)^2)) / (V0(i)+sqrt(2*V0(i))*K(i)+K(i)^2);
            a0=1;
            a1=(2*(K(i)^2-V0(i))) / (V0(i)+sqrt(2*V0(i))*K(i)+K(i)^2);
            a2=(V0(i)-sqrt(2*V0(i))*K(i)+K(i)^2) / (V0(i)+sqrt(2*V0(i))*K(i)+K(i)^2);

            B(i,:)=[b0,b1,b2];
            A(i,:)=[a0,a1,a2];


        elseif Filt(i,2) ==maxFc && V0(i)>0
            % High Shelf Boost
            b0 = (V0(i)+sqrt(2*V0(i))*K(i)+K(i)^2) /(1+sqrt(2)*K(i)+K(i)^2);
            b1= (2*(K(i)^2-V0(i))) / (1+sqrt(2)*K(i)+K(i)^2);
            b2=  (V0(i)-sqrt(2*V0(i))*K(i)+K(i)^2) / (1+sqrt(2)*K(i)+K(i)^2);
            a0=1;
            a1= (2*(K(i)^2-1)) / (1+(sqrt(2)*K(i))+K(i)^2);
            a2= (1-(sqrt(2)*K(i))+K(i)^2) / (1+(sqrt(2)*K(i))+K(i)^2);

            B(i,:)=[b0,b1,b2];
            A(i,:)=[a0,a1,a2];



        elseif Filt(i,2) == maxFc && V0(i)<0
            %High Shelf Cut

            b0=(V0(i)*(1+sqrt(2)*K(i)+K(i)^2)) / (1+sqrt(2*V0(i))*K(i)+V0(i)*K(i)^2);
            b1=(2*V0(i)*(K(i)^2-1)) / (1+sqrt(2*V0(i))*K(i)+V0(i)*K(i)^2);
            b2=(V0(i)*(1-sqrt(2)*K(i)+K(i)^2)) / (1+sqrt(2*V0(i))*K(i)+V0(i)*K(i)^2);
            a0=1;
            a1=(2*(V0(i)*K(i)^2-1)) / (1+sqrt(2*V0(i))*K(i)+V0(i)*K(i)^2);
            a2=(1-sqrt(2*V0(i))*K(i)+V0(i)*K(i)^2) / (1+sqrt(2*V0(i))*K(i)+V0(i)*K(i)^2);



            B(i,:)=[b0,b1,b2];
            A(i,:)=[a0,a1,a2];






        end
    
end

assignin('base', 'B_paramet', B);
assignin('base', 'A_paramet', A);
coeff_flag=2

else

    A= evalin('base', 'A_paramet');
    B = evalin('base', 'B_paramet');

end
%%
%%%%%%%%%%%%%%%%%%%%%%%%%%%%%%%%%%%%%%%%%%%%%%%%%%%%%%%%%%%%%%%%%%%%%%%%%%%%%%%%%%%%%%%%%%%%%%%%%%%%%%%%%%%%%%%%%%%%%%%%%

if isempty(zi_Arr)
zi_Arr=zeros(3,Numband);
end

for n=1:Numband

        
          [y, zi_Arr(:,n)]=myFilter(B(n,:),A(n,:),x,zi_Arr(:,n));
       
        x=y;
       

  
%%
%%%%%%%%%%%%%%%%%%%%%%%%%%%%%%%%%%%%%%%%%%%%%%%%%%%%%%%%%%%%%%%%%%%%%%%%%%%%%%%%%%%%%%%%%%%%%%%%%%%%%%%%%%%%%%%%%%%%%%%
if counter==130
    counter=0;
end

 [H_temp(1:end,n),w] = freqz(B(n,1:end),A(n,1:end));



 H=H.*H_temp(1:end,n);



 f=w/(2*pi)*fs;


        if n==Numband && strcmp(plotFlag, 'on') && counter==1
        figure(1)
        subplot(2,1,1)

        semilogx(f, mag2db(abs(H)));
        xlabel('Frequency (Hz)')
        ylabel('Magnitude (dB)')
        title('Magnitude Response')
        ylim([-4 4])
        xlim([min(f) max(f)])

        xticks([(min(f)+20) 62.5 125 250 500 1000 2000 4000 8000 16000])
        xticklabels({'20','62.5','125','250','500','1000','2000','4K','8K','16K'})

        subplot(2,1,2)
        plot(w, angle(H));
        xlabel('Normalized Frequency (rad/sample)')
        ylabel('Phase (rad)')
        title('Phase Response')


       
        sgtitle('Parametric EQ');
        end


end


end
%%
%%%%%%%%%%%%%%%%%%%%%%%%%%%%%%%%%%%%%%%%%%%%%%%%%%%%%%%%%%%%%%%%%%%%%%%%%%%%%%%%%%%%%%%%%%%%%%%%%%%%%%%%%%%%%%%%%%%%%%%%%%%%%%%%%%%%%%%55

function [y, zf] = myFilter(B, A, x,zi)



count=double(0);
b0=double(B(1));
b1=double(B(2));
b2=double(B(3));
a0=double(A(1));
a1=double(A(2));
a2=double(A(3));


y = ones(length(x),1);

for n = 1:length(x)
    

    y(n) = (b0/a0) * x(n) + zi(1);
    
    zi(1) = (b1/a0) * x(n) + zi(2) - (a1/a0) * y(n);
   
    zi(2) = (b2/a0) * x(n) + zi(3) - (a2/a0) * y(n);
    
count = count+1;
end



zf = zi;

end

== matlab function impedance_subsystem/Subsystem2/MATLAB Function ==
  data: ohms output; f_out output; x input

function [ohms, f_out]=variableResistor(x)

coder.extrinsic('get_param')
coder.extrinsic('xticks')
coder.extrinsic('xticklabels')

persistent endIndex
persistent t
persistent f f_padded
persistent N 
persistent rho c

if isempty(endIndex)
    
    endIndex=1;

end

Sd=         str2double(get_param('a_LS_model/T&S Values', 'W_Sd'))    *1e-4;  %Area of diagphram [m^2]
Bl=      str2double(get_param('a_LS_model/T&S Values', 'W_Bl'));            %The product of magnetic flux density ie Force Factor

SweepDuration=double(0);
SweepStart =str2double(get_param('a_LS_model/Subsystem4', 'SweepStart'));
SweepStop = str2double(get_param('a_LS_model/Subsystem4', 'SweepStop'));
SweepDuration =str2double(get_param('a_LS_model/Subsystem4', 'SweepTime'));



fs=44100;


if isempty(t)

    t = 0:1/fs:SweepDuration-1/fs;
    N=numel(t);    
    f = logspace(log10(SweepStart),log10(SweepStop),N);
    pad_length = 1024 - mod(N, 1024);  % Calculate the number of elements to pad at the end
    f_padded = [f'; ones(pad_length, 1)];  % pad the end of f
    c=344;% speed of sound m/s
    rho=1.2;% density of air [kg/m^3]

end


f_out=zeros(length(x),1);
X_length=length(x);
 

f_out = f_padded(endIndex:(endIndex)+(X_length-1));
endIndex=endIndex+X_length;



w=2*pi*f_out/fs;

r=sqrt(Sd/pi);
k=w/c;
Zc=(rho*c/Sd)*c;
Rar=Zc*(1/4)*(k*r).^2;
Rer=((Bl/Sd)^2)*(1./Rar);

ohms=zeros(size(x));
ohms=Rer;




%%
%%%%%%%%%%%%%%%%%%%%%%%%%%%%%%%%%%%%%%%%%%%%%%%%%%%%%%%%%%%%%%%%%%%%%%%%%%%%%%%%%%%%%%%%%%%%%%%%%%%%%%%%%%%%%%%%%%%%%%%%%%%%%%%%%%%%





end

== matlab function impedance_subsystem/Subsystem3/MATLAB Function ==
  data: x input; ohms output

function ohms=variableResistor(x)

coder.extrinsic('get_param')
coder.extrinsic('xticks')
coder.extrinsic('xticklabels')



persistent endIndex
persistent t
persistent f f_padded
persistent N 
persistent rho c


if isempty(endIndex)
    
    endIndex=1;

end

Sd=      str2double(get_param('a_LS_model/T&S Values', 'T_Sd'))   *1e-4;  %Area of diagphram [m^2]
Bl=      str2double(get_param('a_LS_model/T&S Values', 'T_Bl'));            %The product of magnetic flux density ie Force Factor


SweepDuration=double(0);
SweepStart =str2double(get_param('a_LS_model/Subsystem4', 'SweepStart'));
SweepStop = str2double(get_param('a_LS_model/Subsystem4', 'SweepStop'));
SweepDuration =str2double(get_param('a_LS_model/Subsystem4', 'SweepTime'));



fs=44100;


if isempty(t)

    t = 0:1/fs:SweepDuration-1/fs;
    N=numel(t);    
    f = logspace(log10(SweepStart),log10(SweepStop),N);
    pad_length = 1024 - mod(N, 1024);  % Calculate the number of elements to pad at the end
    f_padded = [f'; ones(pad_length, 1)];  % Zero-pad the end of f_full
    c=344;
    rho=1.2;% density of air [kg/m^3]
    
end


f_out=zeros(length(x),1);
X_length=length(x);
 

f_out = f_padded(endIndex:(endIndex)+(X_length-1));
endIndex=endIndex+X_length;



w=2*pi*f_out/fs;

r=sqrt(Sd/pi);
k=w/c;
Zc=(rho*c/Sd)*c;
Rar=Zc*(1/4)*(k*r).^2;
Rer=((Bl/Sd)^2)*(1./Rar);
ohms=zeros(size(x));
ohms=Rer;




%%
%%%%%%%%%%%%%%%%%%%%%%%%%%%%%%%%%%%%%%%%%%%%%%%%%%%%%%%%%%%%%%%%%%%%%%%%%%%%%%%%%%%%%%%%%%%%%%%%%%%%%%%%%%%%%%%%%%%%%%%%%%%%%%%%%%%%





end

== matlab function impedance_subsystem/Teensy Script/Teensy_Script ==
%% Creates an arduino script that the user copies into the Teensy SDK



function teensyScriptGen

persistent flag

coder.extrinsic('get_param') %coder.entrinsic allows for functions to be surported in simulink that would otherwise not be
coder.extrinsic('evalin')


saveName = get_param('a_LS_model/Teensy Script', 'savename'); %gets save name for script from mask

if isempty(flag) % Script runs just once flag
    flag=1;
end

if flag==1



    A_paramet = evalin('base', 'A_paramet');
    B_paramet = evalin('base', 'B_paramet');

    A_Hi = evalin('base', 'A_High_shel');
    A_Lo = evalin('base', 'A_Low_shel');

    B_Hi = evalin('base', 'B_High_shel');
    B_Lo = evalin('base', 'B_Low_shel');


  a0_1=A_paramet(1,1), a1_1=A_paramet(1,2), a2_1=A_paramet(1,3) , b0_1=B_paramet(1,1) , b1_1=B_paramet(1,2) , b2_1=B_paramet(1,3) ;
  a0_2=A_paramet(2,1) , a1_2=A_paramet(2,2) , a2_2=A_paramet(2,3) , b0_2=B_paramet(2,1) , b1_2=B_paramet(2,2) , b2_2=B_paramet(2,3) ;
  a0_3=A_paramet(3,1) , a1_3=A_paramet(3,2) , a2_3=A_paramet(3,3) , b0_3=B_paramet(3,1) , b1_3=B_paramet(3,2) , b2_3=B_paramet(3,3) ;
  a0_4=A_paramet(4,1) , a1_4=A_paramet(4,2) , a2_4=A_paramet(4,3) , b0_4=B_paramet(4,1) , b1_4=B_paramet(4,2) , b2_4=B_paramet(4,3) ;
  a0_5=A_paramet(5,1), a1_5=A_paramet(5,2) , a2_5=A_paramet(5,3) , b0_5=B_paramet(5,1) , b1_5=B_paramet(5,2) , b2_5=B_paramet(5,3) ;
  a0_6=A_paramet(6,1) , a1_6=A_paramet(6,2) , a2_6=A_paramet(6,3) , b0_6=B_paramet(6,1) , b1_6=B_paramet(6,2) , b2_6=B_paramet(6,3) ;

  a0_Lo=A_Lo(1,1) , a1_Lo=A_Lo(1,2)  , a2_Lo=A_Lo(1,3)  , b0_Lo=B_Lo(1,1)  , b1_Lo=B_Lo(1,2) , b2_Lo=B_Lo(1,3) ;
  a0_Hi=A_Hi(1,1), a1_Hi=A_Hi(1,2) , a2_Hi=A_Hi(1,3), b0_Hi=B_Hi(1,1) , b1_Hi=B_Hi(1,2), b2_Hi=B_Hi(1,3) ;


% Load original script, scripts should be in the same root as simulink
% model
fileID = fopen('teensy_script.txt', 'r');
originalScript = char(fread(fileID, '*char')');
fclose(fileID);




% Replace NaN values 

tempScript = strrep(originalScript, 'a0_1 = nan', sprintf('a0_1 = %.31f', a0_1));
tempScript = strrep(tempScript, 'a1_1 = nan', sprintf('a1_1 = %.31f', a1_1));
tempScript = strrep(tempScript, 'a2_1 = nan', sprintf('a2_1 = %.31f', a2_1));
tempScript = strrep(tempScript, 'b0_1 = nan', sprintf('b0_1 = %.31f', b0_1));
tempScript = strrep(tempScript, 'b1_1 = nan', sprintf('b1_1 = %.31f', b1_1));
tempScript = strrep(tempScript, 'b2_1 = nan', sprintf('b2_1 = %.31f', b2_1));

tempScript = strrep(tempScript, 'a0_2 = nan', sprintf('a0_2 = %.31f', a0_2));
tempScript = strrep(tempScript, 'a1_2 = nan', sprintf('a1_2 = %.31f', a1_2));
tempScript = strrep(tempScript, 'a2_2 = nan', sprintf('a2_2 = %.31f', a2_2));
tempScript = strrep(tempScript, 'b0_2 = nan', sprintf('b0_2 = %.31f', b0_2));
tempScript = strrep(tempScript, 'b1_2 = nan', sprintf('b1_2 = %.31f', b1_2));
tempScript = strrep(tempScript, 'b2_2 = nan', sprintf('b2_2 = %.31f', b2_2));

tempScript = strrep(tempScript, 'a0_3 = nan', sprintf('a0_3 = %.31f', a0_3));
tempScript = strrep(tempScript, 'a1_3 = nan', sprintf('a1_3 = %.31f', a1_3));
tempScript = strrep(tempScript, 'a2_3 = nan', sprintf('a2_3 = %.31f', a2_3));
tempScript = strrep(tempScript, 'b0_3 = nan', sprintf('b0_3 = %.31f', b0_3));
tempScript = strrep(tempScript, 'b1_3 = nan', sprintf('b1_3 = %.31f', b1_3));
tempScript = strrep(tempScript, 'b2_3 = nan', sprintf('b2_3 = %.31f', b2_3));

tempScript = strrep(tempScript, 'a0_4 = nan', sprintf('a0_4 = %.31f', a0_4));
tempScript = strrep(tempScript, 'a1_4 = nan', sprintf('a1_4 = %.31f', a1_4));
tempScript = strrep(tempScript, 'a2_4 = nan', sprintf('a2_4 = %.31f', a2_4));
tempScript = strrep(tempScript, 'b0_4 = nan', sprintf('b0_4 = %.31f', b0_4));
tempScript = strrep(tempScript, 'b1_4 = nan', sprintf('b1_4 = %.31f', b1_4));
tempScript = strrep(tempScript, 'b2_4 = nan', sprintf('b2_4 = %.31f', b2_4));

tempScript = strrep(tempScript, 'a0_5 = nan', sprintf('a0_5 = %.31f', a0_5));
tempScript = strrep(tempScript, 'a1_5 = nan', sprintf('a1_5 = %.31f', a1_5));
tempScript = strrep(tempScript, 'a2_5 = nan', sprintf('a2_5 = %.31f', a2_5));
tempScript = strrep(tempScript, 'b0_5 = nan', sprintf('b0_5 = %.31f', b0_5));
tempScript = strrep(tempScript, 'b1_5 = nan', sprintf('b1_5 = %.31f', b1_5));
tempScript = strrep(tempScript, 'b2_5 = nan', sprintf('b2_5 = %.31f', b2_5));

tempScript = strrep(tempScript, 'a0_6 = nan', sprintf('a0_6 = %.31f', a0_6));
tempScript = strrep(tempScript, 'a1_6 = nan', sprintf('a1_6 = %.31f', a1_6));
tempScript = strrep(tempScript, 'a2_6 = nan', sprintf('a2_6 = %.31f', a2_6));
tempScript = strrep(tempScript, 'b0_6 = nan', sprintf('b0_6 = %.31f', b0_6));
tempScript = strrep(tempScript, 'b1_6 = nan', sprintf('b1_6 = %.31f', b1_6));
tempScript = strrep(tempScript, 'b2_6 = nan', sprintf('b2_6 = %.31f', b2_6));

tempScript = strrep(tempScript, 'a0_Lo = nan', sprintf('a0_Lo = %.31f', a0_Lo));
tempScript = strrep(tempScript, 'a1_Lo = nan', sprintf('a1_Lo = %.31f', a1_Lo));
tempScript = strrep(tempScript, 'a2_Lo = nan', sprintf('a2_Lo = %.31f', a2_Lo));
tempScript = strrep(tempScript, 'b0_Lo = nan', sprintf('b0_Lo = %.31f', b0_Lo));
tempScript = strrep(tempScript, 'b1_Lo = nan', sprintf('b1_Lo = %.31f', b1_Lo));
tempScript = strrep(tempScript, 'b2_Lo = nan', sprintf('b2_Lo = %.31f', b2_Lo));

tempScript = strrep(tempScript, 'a0_Hi = nan', sprintf('a0_Hi = %.31f', a0_Lo));
tempScript = strrep(tempScript, 'a1_Hi = nan', sprintf('a1_Hi = %.31f', a1_Lo));
tempScript = strrep(tempScript, 'a2_Hi = nan', sprintf('a2_Hi = %.31f', a2_Lo));
tempScript = strrep(tempScript, 'b0_Hi = nan', sprintf('b0_Hi = %.31f', b0_Lo));
tempScript = strrep(tempScript, 'b1_Hi = nan', sprintf('b1_Hi = %.31f', b1_Lo));
tempScript = strrep(tempScript, 'b2_Hi = nan', sprintf('b2_Hi = %.31f', b2_Lo));


% Save modified script to new file
fileID = fopen(saveName, 'w');
fwrite(fileID, tempScript, 'char');
fclose(fileID);

flag=2;


end
